simulink model "XY_CL_multi_agent"  (R2023a)
settings: Solver=FixedStepAuto  StartTime=0.0  StopTime=inf  FixedStep=0.01  RelTol=1e-3
model workspace (MAT data in the model file):
  SL_ROS_VariableLengthArrays_MaxSizes.CommonInfo.ArrayTruncateAction = 'EmitWarning'
  SL_ROS_VariableLengthArrays_MaxSizes.MsgTypeMap = containers.Map
  SL_ROS_VariableLengthArrays_MaxSizes.MsgTypeMap.serialization.keys = {'gazebo_msgs/GetModelStateRequest'}
  SL_ROS_VariableLengthArrays_MaxSizes.MsgTypeMap.serialization.values{1}(1).PropertyName = 'ModelName'
  SL_ROS_VariableLengthArrays_MaxSizes.MsgTypeMap.serialization.values{1}(1).DataType = 'uint8'
  SL_ROS_VariableLengthArrays_MaxSizes.MsgTypeMap.serialization.values{1}(1).MaxLength = 6
  SL_ROS_VariableLengthArrays_MaxSizes.MsgTypeMap.serialization.values{1}(2).PropertyName = 'RelativeEntityName'
  SL_ROS_VariableLengthArrays_MaxSizes.MsgTypeMap.serialization.values{1}(2).DataType = 'uint8'
  SL_ROS_VariableLengthArrays_MaxSizes.MsgTypeMap.serialization.values{1}(2).MaxLength = 6
  SL_ROS_VariableLengthArrays_MaxSizes.MsgTypeMap.serialization.uniformity = 0
  SL_ROS_VariableLengthArrays_MaxSizes.MsgTypeMap.serialization.keyType = 'char'
  SL_ROS_VariableLengthArrays_MaxSizes.MsgTypeMap.serialization.valueType = 'any'
undefined symbols (not defined in the file): Angular, Linear
libraries: robotlib x11
settings Model: PacingRate=10  Creator=yoav  LastModifiedBy=connectlab
settings SolverCC: InsertRTBMode=Never (minimum delay)
settings OptimizationCC: EnhancedBackFolding=on  PassReuseOutputArgsAs=Individual arguments  ZeroExternalMemoryAtStartup=off  ZeroInternalMemoryAtStartup=off  MaxStackSize=64  OptimizeBlockOrder=speed  DifferentSizesBufferReuse=on  OptimizationCustomize=off  EfficientTunableParamExpr=on
settings DebuggingCC: ParameterTunabilityLossMsg=error
settings HardwareCC: ProdBitPerPointer=32  ProdBitPerSizeT=32  ProdBitPerPtrDiffT=32  ProdLargestAtomicFloat=None  ProdIntDivRoundTo=Undefined  ProdEndianess=Unspecified  ProdWordSize=32  ProdHWDeviceType=Generic->Unspecified (assume 32-bit Generic)
settings SFSimCC: MATLABDynamicMemAlloc=off
settings RTWCC: Description=Embedded Coder  SystemTargetFile=ert.tlc  HardwareBoard=Robot Operating System (ROS)  TLCOptions="-aInlineSetEventsForThisBaseRateFcn=TLC_FALSE -aSuppressMultiTaskScheduler=TLC_FALSE  -aRateBasedStepFcn=0"  TemplateMakefile=ert_default_tmf  Toolchain=Catkin  TargetLang=C++
settings CodeAppCC: ForceParamTrailComments=on  IgnoreCustomStorageClasses=off  OperatorAnnotations=on  SimulinkDataObjDesc=on  SFDataObjDesc=on  InsertBlockDesc=on
settings ERTTargetCC: ExtMode=on  ExtModeMexArgs='192.168.1.155' 0 17725

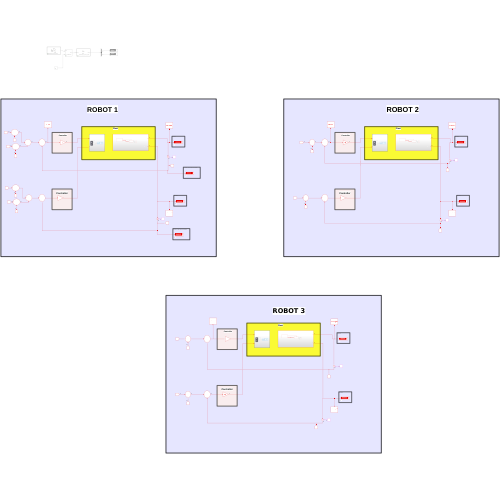
[thumbnail: Simulink's stored preview of the top-level diagram]
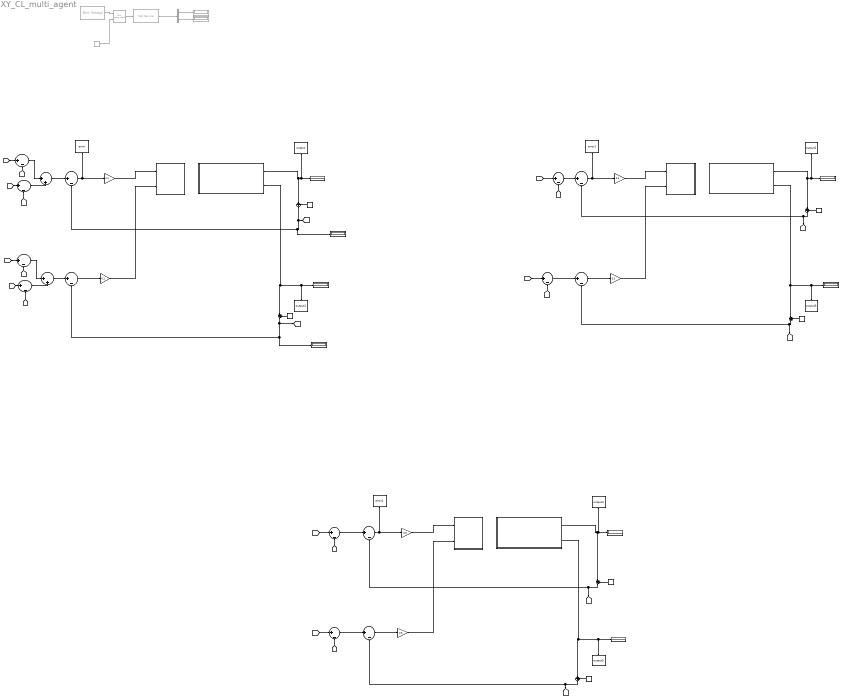
== system XY_CL_multi_agent ==
  note: ROBOT 3
  note: ROBOT 2
  note: ROBOT 1
  note: Controller
  note: Controller
  note: Plant
  note: Position
  note: X
  note: Position
  note: Y
  note: Position
  note: Position
  note: Controller
  note: Plant
  note: Y
  note: Controller
  note: X
  note: Position
  note: Position
  note: Controller
  note: Plant
  note: Y
  note: Controller
  note: X
  note: X
  note: Position after initial condition
  note: Position after initial condition
  note: Y
  Blank Message : robotlib/Blank Message  Commented=on  messageClass=Service Request  entityType=gazebo_msgs/GetModelState  messageType=gazebo_msgs/GetModelStateRequest  SampleTime=inf  legacyBusStruct=off
      settings: LibrarySourceBlock=roslib/ROS/Blank Message
  Bus Assignment : BusAssignment  Commented=on  AssignedSignals=ModelName
  Bus Selector1 : BusSelector  Commented=on  OutputSignals=Pose.Position.X,Pose.Position.Y
  Call Service : robotlib/Call Service  Commented=on  topicSource=Select from ROS network  service=/gazebo/get_model_state  serviceType=gazebo_msgs/GetModelState  connectionTimeout=inf  keepPersistent=on  ShowErrorCodeOutput=off  legacyBusStruct=off
      settings: LibrarySourceBlock=roslib/ROS/Call Service
  Constant : Constant  Value=6
  Constant1 : Constant  Value=2
  Constant2 : Constant  Value=5
  Constant3 : Constant  Value=8
  Constant4 : Constant  Value=2
  Constant5 : Constant  Value=-4
  Constant6 : Constant  Commented=on
  Display : Display  Commented=on
  Display{1..6,8..9} (8 alike) : Display
  Display7 : Display  Commented=on
  Gain1 : Gain  Gain=0.1
  Gain2 : Gain  Gain=0.1
  Gain{3..6} (4 alike) : Gain  Gain=0.5
  Subsystem : Subsystem
  Subsystem1 : Subsystem
  Subsystem2 : Subsystem
  Subsystem3 : Subsystem
  Subsystem4 : Subsystem
  Subsystem5 : Subsystem
  Sum{,1..5,7..8,10..16} (15 alike) : Sum  Inputs=|+-
  Sum{6,9,17..21} (7 alike) : Sum  Inputs=|++
  To Workspace : ToWorkspace  VariableName=error  SaveFormat=Timeseries  SampleTime=-1
  To Workspace1 : ToWorkspace  VariableName=output  SaveFormat=Timeseries  SampleTime=-1
  To Workspace2 : ToWorkspace  VariableName=output1  SaveFormat=Timeseries  SampleTime=-1
  To Workspace3 : ToWorkspace  VariableName=error1  SaveFormat=Timeseries  SampleTime=-1
  To Workspace4 : ToWorkspace  VariableName=output2  SaveFormat=Timeseries  SampleTime=-1
  To Workspace5 : ToWorkspace  VariableName=output3  SaveFormat=Timeseries  SampleTime=-1
  To Workspace6 : ToWorkspace  VariableName=error2  SaveFormat=Timeseries  SampleTime=-1
  To Workspace7 : ToWorkspace  VariableName=output4  SaveFormat=Timeseries  SampleTime=-1
  To Workspace8 : ToWorkspace  VariableName=output5  SaveFormat=Timeseries  SampleTime=-1
  wires:
  Subsystem1/1(Output) -> Sum16/1, Display3/1, To Workspace1/1
  Sum6/1 -> Sum/1
  Sum/1 -> To Workspace/1, Gain1/1
  Gain1/1 -> Subsystem/1(In1)
  Sum9/1 -> Sum1/1
  Sum1/1 -> Gain2/1
  Gain2/1 -> Subsystem/2(In2)
  Subsystem1/2(Out1) -> Display1/1, To Workspace2/1, Sum17/1
  Sum12/1 -> Sum2/1
  Sum3/1 -> Gain4/1
  Subsystem3/1(Out4) -> Sum18/1, Display4/1, To Workspace4/1
  Sum2/1 -> To Workspace3/1, Gain3/1
  Sum13/1 -> Sum3/1
  Gain3/1 -> Subsystem2/1(In1)
  Gain4/1 -> Subsystem2/2(In2)
  Subsystem3/2(Out1) -> Sum19/1, Display2/1, To Workspace5/1
  Sum14/1 -> Sum4/1
  Sum5/1 -> Gain6/1
  Subsystem5/1(Out4) -> Sum20/1, Display6/1, To Workspace7/1
  Sum4/1 -> To Workspace6/1, Gain5/1
  Sum15/1 -> Sum5/1
  Gain5/1 -> Subsystem4/1(In1)
  Gain6/1 -> Subsystem4/2(In2)
  Subsystem5/2(Out1) -> Sum21/1, Display5/1, To Workspace8/1
  Sum8/1 -> Sum6/2
  Sum7/1 -> Sum6/1
  [X2] -> Sum7/1
  [X1] -> Sum7/2
  [X1] -> Sum8/2
  [X3] -> Sum8/1
  [Y1] -> Sum11/2
  Sum11/1 -> Sum9/2
  Sum10/1 -> Sum9/1
  [Y2] -> Sum10/1
  [Y3] -> Sum11/1
  [Y1] -> Sum10/2
  [X1] -> Sum12/1
  [X2] -> Sum12/2
  [Y1] -> Sum13/1
  [Y2] -> Sum13/2
  [X1] -> Sum14/1
  [X3] -> Sum14/2
  [Y1] -> Sum15/1
  [Y3] -> Sum15/2
  Bus Selector1/2 -> Display7/1  "<Y>"
  Bus Selector1/1 -> Display/1  "<X>"
  Call Service/1 -> Bus Selector1/1
  Blank Message/1 -> Bus Assignment/1
  Bus Assignment/1 -> Call Service/1
  Constant6/1 -> Bus Assignment/2
  Constant/1 -> Sum16/2
  Sum16/1 -> [X1], Display8/1, Sum/2
  Sum17/1 -> [Y1], Display9/1, Sum1/2
  Constant1/1 -> Sum17/2
  Constant2/1 -> Sum18/2
  Sum18/1 -> [X2], Sum2/2
  Constant3/1 -> Sum19/2
  Sum19/1 -> [Y2], Sum3/2
  Constant4/1 -> Sum20/2
  Sum20/1 -> Sum4/2, [X3]
  Constant5/1 -> Sum21/2
  Sum21/1 -> Sum5/2, [Y3]

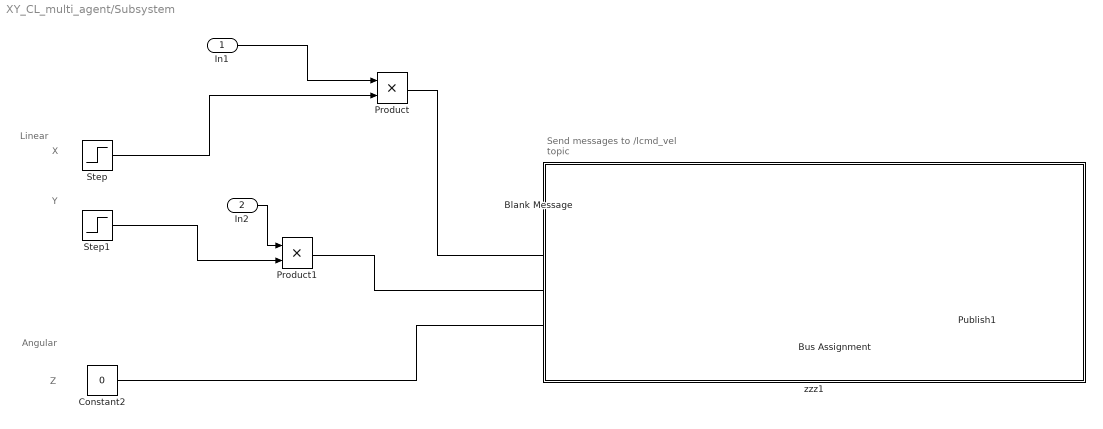
== system XY_CL_multi_agent/Subsystem ==
  note: Send messages to /lcmd_vel topic
  note: Y
  note: X
  note: Linear
  note: Angular
  note: Z
  In1 : Inport
  In2 : Inport  Port=2
  Blank Message : robotlib/Blank Message  messageClass=Message  entityType=geometry_msgs/Twist  messageType=geometry_msgs/Twist  SampleTime=inf  legacyBusStruct=off
  Bus Assignment : BusAssignment  AssignedSignals=Linear.X,Linear.Y,Angular.Z
  Constant2 : Constant  Value=0
  Product : Product
  Product1 : Product
  Publish1 : robotlib/Publish  topicSource=Specify your own  topic=/robot1/cmd_vel  messageType=geometry_msgs/Twist  legacyBusStruct=off  messageQueueLength=105
  Step : Step  Time=0  SampleTime=0
  Step1 : Step  Time=0  SampleTime=0
  zzz1 : Subsystem  TreatAsAtomicUnit=on
      settings: OpenFcn=% no-op
      mask Display: disp('')
  wires:
  Blank Message/1 -> Bus Assignment/1
  Bus Assignment/1 -> Publish1/1
  Constant2/1 -> Bus Assignment/4
  In1/1 -> Product/1
  Step/1 -> Product/2
  Product/1 -> Bus Assignment/2
  Step1/1 -> Product1/2
  In2/1 -> Product1/1
  Product1/1 -> Bus Assignment/3

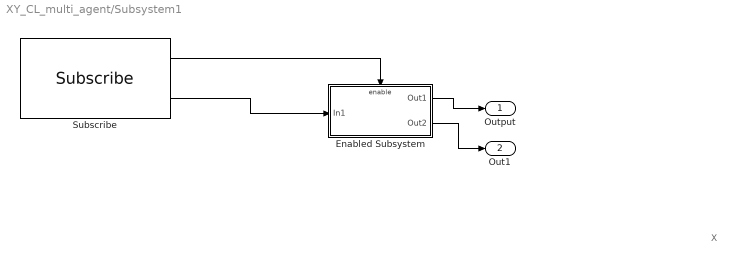
== system XY_CL_multi_agent/Subsystem1 ==
  note: X
  Enabled Subsystem : Subsystem  TreatAsAtomicUnit=on
  Subscribe : robotlib/Subscribe  topicSource=Select from ROS network  topic=/robot1/odom  messageType=nav_msgs/Odometry  SampleTime=-1  legacyBusStruct=off  messageQueueLength=1
      settings: LibrarySourceBlock=roslib/ROS/Subscribe
  Output : Outport
  Out1 : Outport  Port=2
  wires:
  Subscribe/2 -> Enabled Subsystem/1(In1)
  Subscribe/1 -> Enabled Subsystem/Enable
  Enabled Subsystem/1(Out1) -> Output/1
  Enabled Subsystem/2(Out2) -> Out1/1

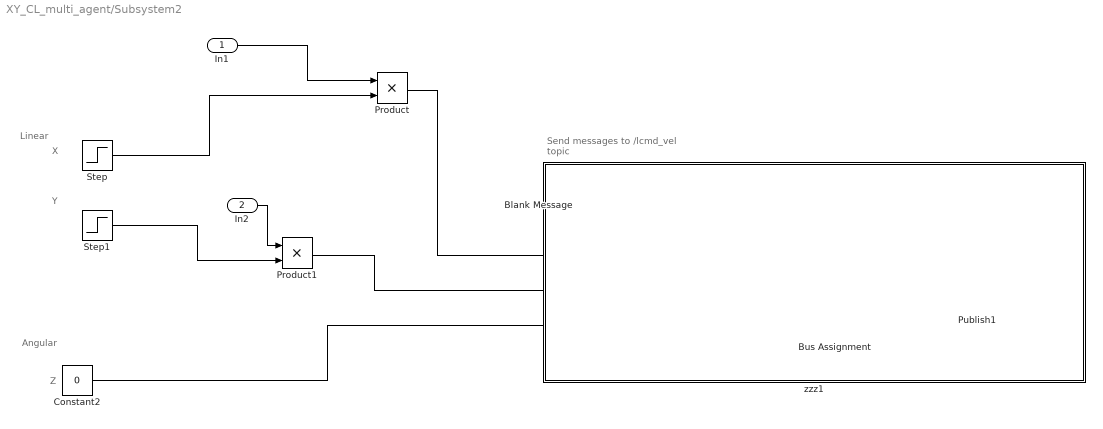
== system XY_CL_multi_agent/Subsystem2 ==
  note: Send messages to /lcmd_vel topic
  note: Y
  note: X
  note: Linear
  note: Angular
  note: Z
  In1 : Inport
  In2 : Inport  Port=2
  Blank Message : robotlib/Blank Message  messageClass=Message  entityType=geometry_msgs/Twist  messageType=geometry_msgs/Twist  SampleTime=inf  legacyBusStruct=off
  Bus Assignment : BusAssignment  AssignedSignals=Linear.X,Linear.Y,Angular.Z
  Constant2 : Constant  Value=0
  Product : Product
  Product1 : Product
  Publish1 : robotlib/Publish  topicSource=Specify your own  topic=/robot2/cmd_vel  messageType=geometry_msgs/Twist  legacyBusStruct=off  messageQueueLength=105
  Step : Step  Time=0  SampleTime=0
  Step1 : Step  Time=0  SampleTime=0
  zzz1 : Subsystem  TreatAsAtomicUnit=on
      settings: OpenFcn=% no-op
      mask Display: disp('')
  wires:
  Blank Message/1 -> Bus Assignment/1
  Bus Assignment/1 -> Publish1/1
  Constant2/1 -> Bus Assignment/4
  In1/1 -> Product/1
  Step/1 -> Product/2
  Product/1 -> Bus Assignment/2
  Step1/1 -> Product1/2
  In2/1 -> Product1/1
  Product1/1 -> Bus Assignment/3

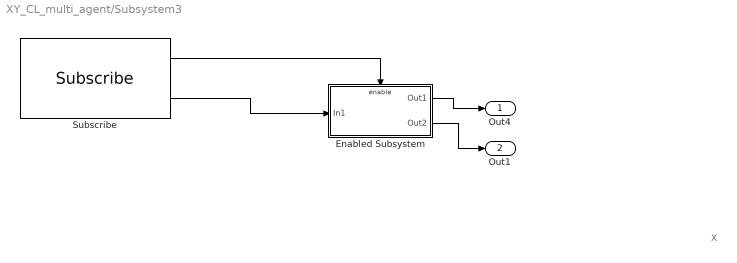
== system XY_CL_multi_agent/Subsystem3 ==
  note: X
  Enabled Subsystem : Subsystem  TreatAsAtomicUnit=on
  Subscribe : robotlib/Subscribe  topicSource=Select from ROS network  topic=/robot2/odom  messageType=nav_msgs/Odometry  SampleTime=-1  legacyBusStruct=off  messageQueueLength=1
      settings: LibrarySourceBlock=roslib/ROS/Subscribe
  Out4 : Outport
  Out1 : Outport  Port=2
  wires:
  Subscribe/2 -> Enabled Subsystem/1(In1)
  Subscribe/1 -> Enabled Subsystem/Enable
  Enabled Subsystem/1(Out1) -> Out4/1
  Enabled Subsystem/2(Out2) -> Out1/1

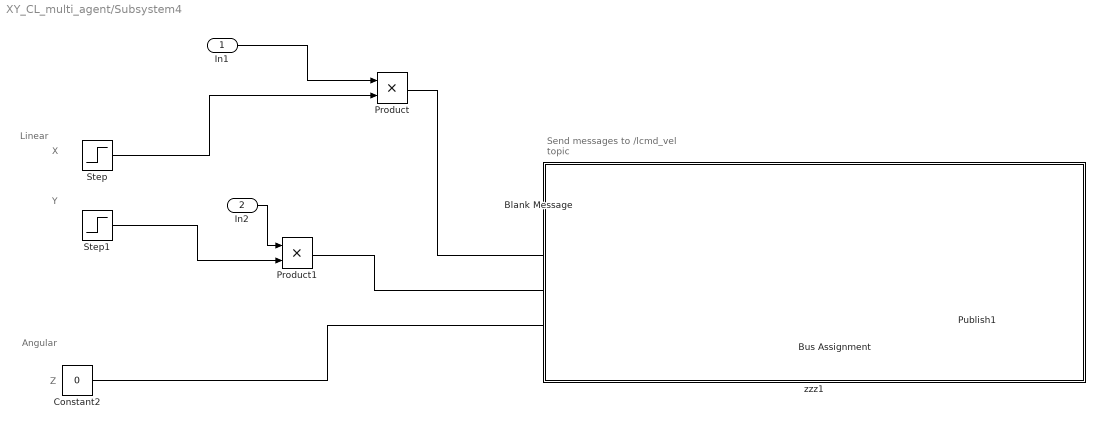
== system XY_CL_multi_agent/Subsystem4 ==
  note: Send messages to /lcmd_vel topic
  note: Y
  note: X
  note: Linear
  note: Angular
  note: Z
  In1 : Inport
  In2 : Inport  Port=2
  Blank Message : robotlib/Blank Message  messageClass=Message  entityType=geometry_msgs/Twist  messageType=geometry_msgs/Twist  SampleTime=inf  legacyBusStruct=off
  Bus Assignment : BusAssignment  AssignedSignals=Linear.X,Linear.Y,Angular.Z
  Constant2 : Constant  Value=0
  Product : Product
  Product1 : Product
  Publish1 : robotlib/Publish  topicSource=Specify your own  topic=/robot3/cmd_vel  messageType=geometry_msgs/Twist  legacyBusStruct=off  messageQueueLength=105
  Step : Step  Time=0  SampleTime=0
  Step1 : Step  Time=0  SampleTime=0
  zzz1 : Subsystem  TreatAsAtomicUnit=on
      settings: OpenFcn=% no-op
      mask Display: disp('')
  wires:
  Blank Message/1 -> Bus Assignment/1
  Bus Assignment/1 -> Publish1/1
  Constant2/1 -> Bus Assignment/4
  In1/1 -> Product/1
  Step/1 -> Product/2
  Product/1 -> Bus Assignment/2
  Step1/1 -> Product1/2
  In2/1 -> Product1/1
  Product1/1 -> Bus Assignment/3

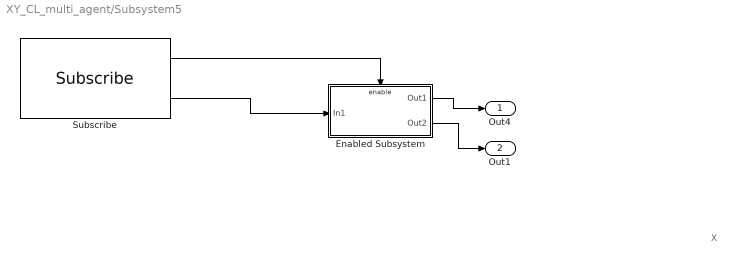
== system XY_CL_multi_agent/Subsystem5 ==
  note: X
  Enabled Subsystem : Subsystem  TreatAsAtomicUnit=on
  Subscribe : robotlib/Subscribe  topicSource=Select from ROS network  topic=/robot3/odom  messageType=nav_msgs/Odometry  SampleTime=-1  legacyBusStruct=off  messageQueueLength=1
      settings: LibrarySourceBlock=roslib/ROS/Subscribe
  Out4 : Outport
  Out1 : Outport  Port=2
  wires:
  Subscribe/2 -> Enabled Subsystem/1(In1)
  Subscribe/1 -> Enabled Subsystem/Enable
  Enabled Subsystem/1(Out1) -> Out4/1
  Enabled Subsystem/2(Out2) -> Out1/1

== system XY_CL_multi_agent/Subsystem/zzz1 ==

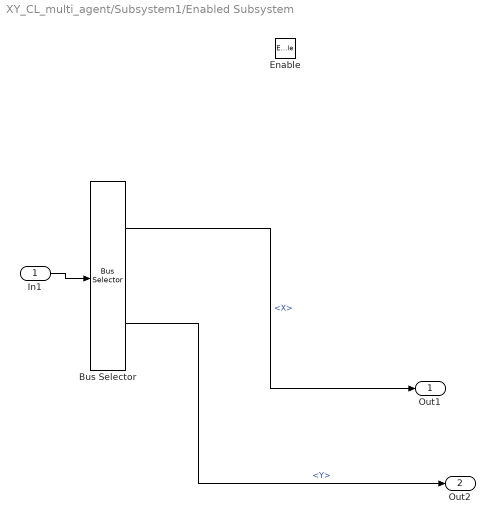
== system XY_CL_multi_agent/Subsystem1/Enabled Subsystem ==
  In1 : Inport
  Enable : EnablePort
  Bus Selector : BusSelector  OutputSignals=Pose.Pose.Position.X,Pose.Pose.Position.Y
  Out1 : Outport
  Out2 : Outport  Port=2
  wires:
  In1/1 -> Bus Selector/1
  Bus Selector/1 -> Out1/1  "<X>"
  Bus Selector/2 -> Out2/1  "<Y>"

== system XY_CL_multi_agent/Subsystem2/zzz1 ==

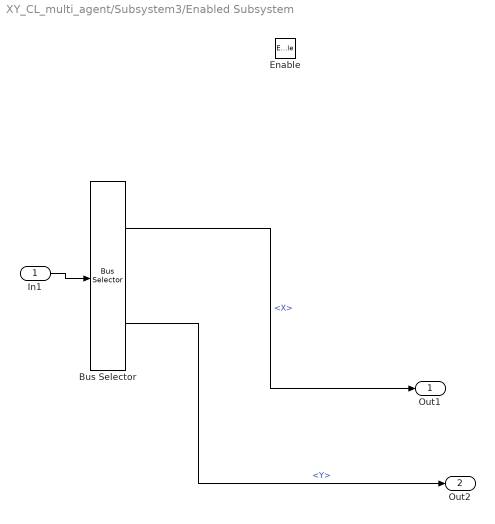
== system XY_CL_multi_agent/Subsystem3/Enabled Subsystem ==
  In1 : Inport
  Enable : EnablePort
  Bus Selector : BusSelector  OutputSignals=Pose.Pose.Position.X,Pose.Pose.Position.Y
  Out1 : Outport
  Out2 : Outport  Port=2
  wires:
  In1/1 -> Bus Selector/1
  Bus Selector/1 -> Out1/1  "<X>"
  Bus Selector/2 -> Out2/1  "<Y>"

== system XY_CL_multi_agent/Subsystem4/zzz1 ==

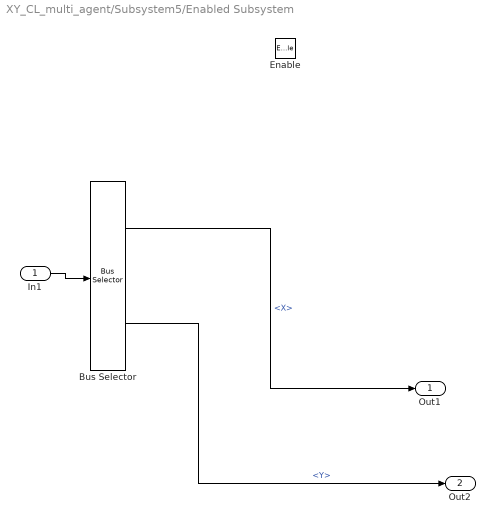
== system XY_CL_multi_agent/Subsystem5/Enabled Subsystem ==
  In1 : Inport
  Enable : EnablePort
  Bus Selector : BusSelector  OutputSignals=Pose.Pose.Position.X,Pose.Pose.Position.Y
  Out1 : Outport
  Out2 : Outport  Port=2
  wires:
  In1/1 -> Bus Selector/1
  Bus Selector/1 -> Out1/1  "<X>"
  Bus Selector/2 -> Out2/1  "<Y>"
